simulink model "SOS_Gen3_Compressor_Master"  (R2026a)
settings: Solver=ode1  StopTime=inf  FixedStep=0.003
libraries: dspstat3 x1
(part 2 of 2)

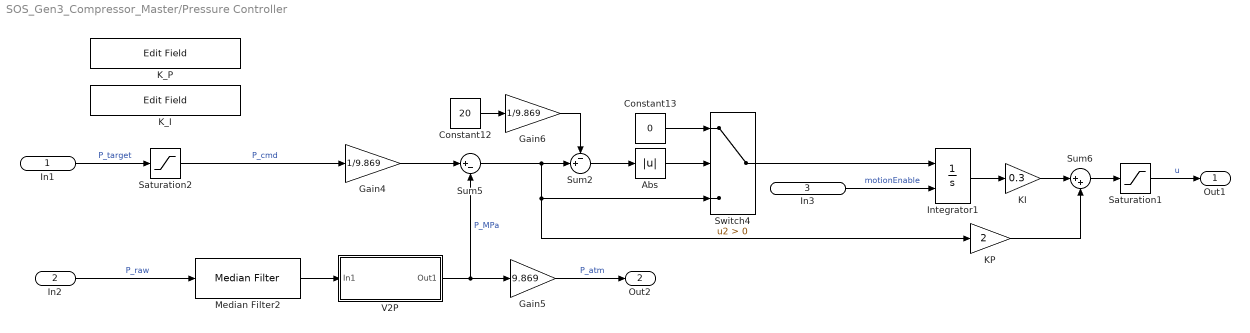
== system SOS_Gen3_Compressor_Master/Pressure Controller ==
  In1 : Inport
  In2 : Inport  Port=2
  In3 : Inport  Port=3
  Abs : Abs  SaturateOnIntegerOverflow=off
  Constant12 : Constant  Value=20
  Constant13 : Constant  Value=0
  Gain4 : Gain  Gain=1/9.869
  Gain5 : Gain  Gain=9.869
  Gain6 : Gain  Gain=1/9.869
  Integrator1 : Integrator  ExternalReset=either
  KI : Gain  Gain=0.3
  KP : Gain  Gain=2
  K_I : EditField  LabelPosition=Hide  ShowInitialText=on  Alignment=Center
  K_P : EditField  LabelPosition=Hide  ShowInitialText=on  Alignment=Center
  Median Filter2 : dspstat3/Median Filter  WindowLength=7  SimulateUsing=Interpreted execution
      settings: LibrarySourceBlock=|
      | dspfdesign/Median
      | Filter
  Saturation1 : Saturate  UpperLimit=10  LowerLimit=-10
  Saturation2 : Saturate  UpperLimit=100  LowerLimit=5
  Sum2 : Sum  Inputs=-+|
  Sum5 : Sum  Inputs=|+-
  Sum6 : Sum  Inputs=|++
  Switch4 : Switch  Criteria=u2 > Threshold  SaturateOnIntegerOverflow=off  InputSameDT=off
  V2P : Subsystem
  Out1 : Outport
  Out2 : Outport  Port=2
  wires:
  Saturation1/1 -> Out1/1  "u"
  Abs/1 -> Switch4/2
  Gain4/1 -> Sum5/1
  Median Filter2/1 -> V2P/1(In1)
  Switch4/1 -> Integrator1/1
  KP/1 -> Sum6/2
  In3/1 -> Integrator1/2  "motionEnable"
  Gain5/1 -> Out2/1  "P_atm"
  KI/1 -> Sum6/1
  Saturation2/1 -> Gain4/1  "P_cmd"
  Constant13/1 -> Switch4/1
  Constant12/1 -> Gain6/1
  Sum5/1 -> Sum2/2, KP/1, Switch4/3
  In2/1 -> Median Filter2/1  "P_raw"
  Integrator1/1 -> KI/1
  V2P/1(Out1) -> Gain5/1, Sum5/2  "P_MPa"
  Sum2/1 -> Abs/1
  Sum6/1 -> Saturation1/1
  Gain6/1 -> Sum2/1
  In1/1 -> Saturation2/1  "P_target"

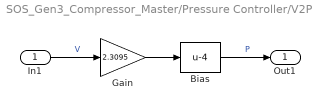
== system SOS_Gen3_Compressor_Master/Pressure Controller/V2P ==
  In1 : Inport
  Bias : Bias  Bias=-4  SaturateOnIntegerOverflow=off
  Gain : Gain  Gain=2.3095
  Out1 : Outport
  wires:
  In1/1 -> Gain/1  "V"
  Bias/1 -> Out1/1  "P"
  Gain/1 -> Bias/1

== matlab function SOS_Gen3_Compressor_Master/MATLAB Function ==
  data: u input; y output
function y = latch(u)

persistent latchedValue

if isempty(latchedValue)
    latchedValue = 0;
end

if u ~= -1
    latchedValue = u;
end

y = latchedValue;

== stateflow chart SOS_Gen3_Compressor_Master/StateDiagram ==
  state Homing_Required
    during:
    confirmedMode = modeConfBit2*4 + modeConfBit1*2+modeConfBit0;
    state Init
      entry:
      modeBit0 = 0;
      modeBit1 = 0;
      modeBit2 = 0;
      motionEnable = 0;
      faultReset = 0;
      statusCode = 0;
    state Request_Homing
      entry:
      modeBit0 = 1;
      modeBit1 = 0;
      modeBit2 = 1;
      requestedMode = 5;
    state Homing
      entry:
      motionEnable = 1;
      statusCode = 1;
    (default) -> Init
    Init -> Request_Homing : [appRequestedMode == 1]
    Request_Homing -> Homing : [requestedMode == confirmedMode && after(100,msec)]
  state Fault_Active
    exit:
    faultReset = 0;
    state Safe
      entry:
      modeBit0 = 0;
      modeBit1 = 0;
      modeBit2 = 0;
      motionEnable = 0;
      faultReset = 0;
      statusCode = 0;
    state Mirror
      entry:
      modeBit0 = modeConfBit0;
      modeBit1 = modeConfBit1;
      modeBit2 = modeConfBit2;
    state Pulse_Reset
      entry:
      faultReset = 1;
    (default) -> Safe
    Safe -> Mirror : [after(100,msec)]
    Mirror -> Pulse_Reset : [appRequestedMode == 5]
  note: Status Codes
      | Code
      | Status
      |
      | 0
      | Idle
      |
      | 1
      | Homing
      |
      | 2
      | Position Control
      |
      | 3
      | Velocity Control
      |
      | 4
      | Pressure Control
  state Normal
    during:
    confirmedMode = modeConfBit2*4 + modeConfBit1*2+modeConfBit0;
    state Idle
      entry:
      modeBit0 = 0;
      modeBit1 = 0;
      modeBit2 = 0;
      motionEnable = 0;
      faultReset = 0;
      statusCode = 0;
    state Position_Control
      entry:
      positionMargin = 0.5; % mm
      exit:
      voltageOut = 0;
      state Request_Position_Control
        entry:
        modeBit0 = 1;
        modeBit1 = 1;
        modeBit2 = 0;
        requestedMode = 3;
      state Estimate_Position
        entry:
        statusCode = 2;
        counter = 0;
        buffer = zeros(3,1);
        during:
        counter = counter+1;
        buffer(counter) = position;
        exit:
        medianPosition = median(buffer);
      state Move_Up
        entry:
        counter = 0;
        voltageOut = 10;
        motionEnable = 1
        during:
        if position >= targetPosition-positionMargin
        counter = min(counter+1,3);
        else
        counter = max(counter-1,0)
        end
      state Move_Down
        entry:
        counter = 0;
        voltageOut = -10;
        motionEnable = 1;
        during:
        if position <= targetPosition+positionMargin
        counter = min(counter+1,3);
        else
        counter = max(counter-1,0)
        end
      state Hold_Position
        entry:
        statusCode = 2.1;
        counter = 0;
        voltageOut = 0;
        during:
        if abs(position-targetPosition) > positionMargin
        counter = counter + 1;
        else
        counter = max(counter-1,0);
        end
      (default) -> Request_Position_Control
      Request_Position_Control -> Estimate_Position : [confirmedMode == requestedMode & after(100,msec)]
      Hold_Position -> Estimate_Position : [counter >= 3]
      Estimate_Position -> (junction 95) : [counter >= 3]
      (junction 95) -> Move_Up [order 2] : [medianPosition < targetPosition-positionMargin]
      (junction 95) -> Hold_Position [order 3] : [abs(position-targetPosition) <= positionMargin]
      (junction 95) -> Move_Down [order 1] : [medianPosition > targetPosition+positionMargin]
      Move_Up -> Hold_Position : [counter >= 3]
      Move_Down -> Hold_Position : [counter >= 3]
    state Request_Velocity_Control
      entry:
      modeBit0 = 1;
      modeBit1 = 1;
      modeBit2 = 0;
      requestedMode = 3;
    state Velocity_Control
      entry:
      statusCode = 3;
      voltageOut = targetVelocity*(10/3);
      motionEnable = 1;
      during:
      voltageOut = targetVelocity*(10/3);
      exit:
      motionEnable = 0;
    state Pressure_Control
      entry:
      statusCode = 4;
      useControllerVoltage = 1;
      motionEnable = 1;
      exit:
      useControllerVoltage = 0;
    state Request_Pressure_Control
      entry:
      modeBit0 = 1;
      modeBit1 = 1;
      modeBit2 = 0;
      requestedMode = 3;
    (default) -> Idle
    (junction 114) -> Idle
    (junction 111) -> (junction 114)
    Position_Control -> Idle : [appRequestedMode ~= 2]
    Idle -> (junction 52)
    (junction 52) -> Position_Control [order 1] : [appRequestedMode == 2]
    (junction 52) -> (junction 53) [order 2]
    (junction 53) -> Request_Velocity_Control [order 1] : [appRequestedMode == 3]
    (junction 53) -> (junction 54) [order 2]
    Request_Velocity_Control -> Velocity_Control : [confirmedMode == requestedMode & after(100,msec)]
    Velocity_Control -> (junction 111) : [appRequestedMode ~= 3]
    Pressure_Control -> (junction 111) : [appRequestedMode ~= 4]
    (junction 54) -> Request_Pressure_Control : [appRequestedMode == 4]
    Request_Pressure_Control -> Pressure_Control : [confirmedMode == requestedMode & after(100,msec)]
  (default) -> Homing_Required
  Homing_Required -> Fault_Active [order 2] : [faultActive == 1]
  (junction 119) -> Homing_Required [order 1] : [homingComplete == 0]
  Fault_Active -> (junction 119) : [faultActive == 1]
  (junction 119) -> Normal [order 2] : [homingComplete == 1]
  Normal -> Fault_Active [order 2] : [faultActive == 1]
  Homing_Required -> Normal [order 1] : [homingComplete == 1]
  Normal -> Homing_Required [order 1] : [homingComplete == 0]
  data: appRequestedMode input; modeBit0 output; modeBit1 output; modeBit2 output; motionEnable output; homingComplete input; faultReset output; modeConfBit0 input; modeConfBit1 input; modeConfBit2 input; confirmedMode local; requestedMode local; statusCode output; counter local; buffer local; position input; medianPosition local; targetPosition input; voltageOut output; positionMargin local; useControllerVoltage output; targetVelocity input; faultActive input

== matlab function SOS_Gen3_Compressor_Master/MATLAB Function1 ==
  data: u input; y output
function y = latch(u)

persistent latchedValue

if isempty(latchedValue)
    latchedValue = 0;
end

if u ~= 0
    latchedValue = u;
end

y = latchedValue;
